simulink model "zaddom"  (R2021a)
settings: Solver=VariableStepAuto  StartTime=0.0  StopTime=3  RelTol=1e-3
libraries: simulink x1
settings Model: Creator=sm46651  LastModifiedBy=sm46651

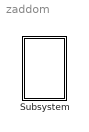
== system zaddom ==
  Subsystem : Subsystem  mask{v0=10, g=9.81, h0=0}

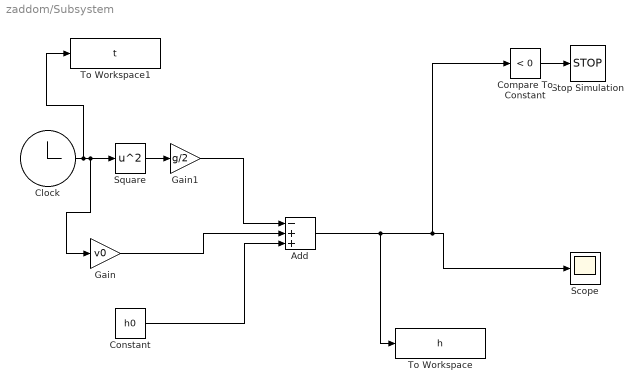
== system zaddom/Subsystem ==
  Add : Sum  Inputs=-++
  Clock : Clock
  Compare To Constant : simulink/Logic and Bit Operations/Compare To Constant  relop=<  const=0  OutDataTypeStr=boolean
  Constant : Constant  Value=h0
  Gain : Gain  Gain=v0
  Gain1 : Gain  Gain=g/2
  Scope : Scope
  Square : Math  Operator=square  SaturateOnIntegerOverflow=on
  Stop Simulation : Stop
  To Workspace : ToWorkspace  VariableName=h  SampleTime=-1
  To Workspace1 : ToWorkspace  VariableName=t  SampleTime=-1
  wires:
  Clock/1 -> To Workspace1/1, Gain/1, Square/1
  Gain/1 -> Add/2
  Square/1 -> Gain1/1
  Constant/1 -> Add/3
  Compare To Constant/1 -> Stop Simulation/1
  Add/1 -> To Workspace/1, Compare To Constant/1, Scope/1
  Gain1/1 -> Add/1
